simulink model "PLL_fault_no_switching"  (R2022a)
settings: Solver=FixedStepAuto  StartTime=0.0  StopTime=1  FixedStep=Ts  RelTol=1e-3
values from neighbouring files (symbols this model uses):
  C_dc = 2.25    [PLLpara.m]
  Cf1 = 0.01    [PLLpara.m]
  Cf2 = 0.01    [PLLpara.m]
  dt_sag = t_c    [GFMPara.m]    (also in GFMPara_exp.m; PLLpara.m; VFMPara.m; VFMPara_exp.m)
  f_switching = 20e3    (= 20000)    [GFMPara_exp.m]    (also in PLLpara.m = 10000; VFMPara_exp.m)
  Id0 = Id    [PLLpara.m]
  Iq02 = (Ug*cos(asin((Xg*Id+Rg*Iq)/Ug))+Id*Rg-Iq*Xg)*Cf2+Iq    [PLLpara.m]
  ki_pll1 = ki    [PLLpara.m]
  kp_pll1 = kp    [PLLpara.m]
  Lc = 1e-9    (= 1e-09)    [GFMPara.m]    (also in GFMPara_exp.m; PLLpara.m; VFMPara.m; VFMPara_exp.m)
  Lf = 0.0592    [GFMPara.m]    (also in GFMPara_exp.m; PLLpara.m = 0.05; VFMPara.m = 0.05; VFMPara_exp.m = 0.05)
  Lg1 = X1    [PLLpara.m]    (also in VFMPara.m; VFMPara_exp.m)
  Lgg = Xgg    [PLLpara.m]    (also in VFMPara.m; VFMPara_exp.m)
  Rf = 1e-3    (= 0.001)    [PLLpara.m]
  Rg1 = R1    [PLLpara.m]    (also in VFMPara.m; VFMPara_exp.m = 4*R1/5)
  Rgg = Rgg    [PLLpara.m]    (also in VFMPara.m; VFMPara_exp.m)
  Sbase = 1    [GFMPara.m]    (also in GFMPara_exp.m; PLLpara.m; VFMPara.m; VFMPara_exp.m)
  t0 = t_sim_start +t_start    [PLLpara.m]    (also in VFMPara_exp.m)
  t0_sag = t_sim_start +t_start    [GFMPara.m]    (also in GFMPara_exp.m; PLLpara.m = 20; VFMPara.m; VFMPara_exp.m = 20)
  Tc = 1/f_switching    (= 5e-05)    [GFMPara_exp.m]    (also in PLLpara.m = 0.0001; VFMPara_exp.m)
  tc = t_c    [PLLpara.m]    (also in VFMPara_exp.m)
  Ts = 1/Fs    (= 1e-05)    [GFMPara.m]    (also in GFMPara_exp.m = 1e-06; PLLpara.m = 1e-06; VFMPara.m = 5e-06; VFMPara_exp.m = 1e-06)
  v_sag = Ug_fault    [GFMPara.m]    (also in GFMPara_exp.m; PLLpara.m; VFMPara.m; VFMPara_exp.m)
  Vbase = 1    [GFMPara.m]    (also in GFMPara_exp.m; PLLpara.m; VFMPara.m; VFMPara_exp.m)
  Vdc = 2.5    [PLLpara.m]
  w_i_GFL1 = 3000 *2*pi    (= 18849.5559215)    [PLLpara.m]
  w_i_GFL2 = 1100 *2*pi    (= 6911.5038379)    [PLLpara.m]
  w_pll1 = 10 *2*pi    (= 62.8318530718)    [PLLpara.m]
  w_tau1 = 1500 *2*pi    (= 9424.77796077)    [PLLpara.m]
  Wbase = 2*pi*50    (= 314.159265359)    [GFMPara.m]    (also in GFMPara_exp.m; PLLpara.m; VFMPara.m; VFMPara_exp.m)
  Zbase = Vbase/Ibase    (= 1)    [GFMPara.m]    (also in GFMPara_exp.m; PLLpara.m; VFMPara.m; VFMPara_exp.m)
undefined symbols (not defined in the file or in its folder): DiscIntNeverNeededParam, Id, initial, Iq, position, postfault_SEP, w_max, w_min, Ws
libraries: spsVoltageMeasurementLib x52, spsCurrentMeasurementLib x48, spsThreePhaseSeriesRLCBranchLib x13, spsControlledVoltageSourceLib x12, powerlib_extras x12, spsIdealSwitchLib x12, spsSeriesRLCBranchLib x7, spsThreePhaseBreakerLib x4, spsHalfBridgeConverterLib x3, spsDCVoltageSourceLib x2, spsThreePhaseFaultLib x2, cstblocks x1
(part 2 of 4)

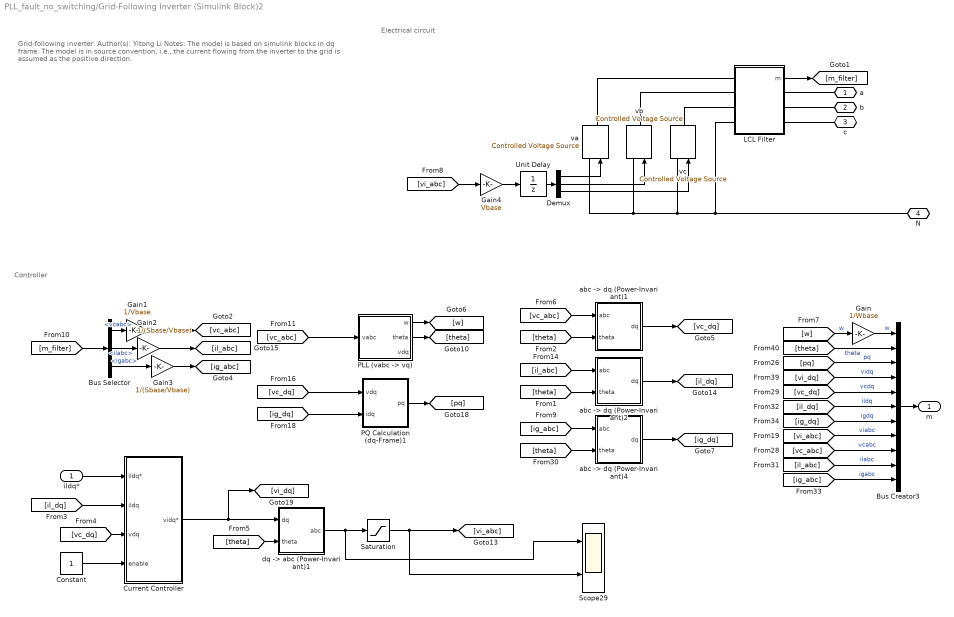
== system PLL_fault_no_switching/Grid-Following Inverter (Simulink Block)2 ==
  note: Grid-following inverter.
      |
      | Author(s): Yitong Li
      |
      | Notes:
      |
      | The model is based on simulink blocks in dq frame.
      |
      | The model is in source convention, i.e., the current flowing from the inverter to the grid is assumed as the positive direction.
  note: Electrical circuit
  note: Controller
  ildq* : Inport
  Bus Creator3 : BusCreator  Inputs=11
  Bus Selector : BusSelector  OutputSignals=vcabc,ilabc,igabc
  Constant : Constant
  Current Controller : Subsystem  mask{Ts=Ts, Wbase=Wbase, Lf=Lf/Wbase, Kg=0, Kp=w_i*Lf/Wbase, Ki=w_i*w_i/4*Lf/Wbase, vdmax=inf, vqmax=inf, Kcd=0}
      mask prompts: Ts "Sampling Time (s)"; Wbase "Base Angular Frequency (rad/s)"; Lf "Inductance"; Kg "Estimator Gain"; Kp "Proportional Gain"; Ki "Integral Gain"; vdmax "Voltage D Limit"; vqmax "Voltage Q Limit"; Kcd "Cross Decoupling Gain"
  Demux : Demux  Outputs=3
  Gain : Gain  Gain=1/Wbase
  Gain1 : Gain  Gain=1/Vbase
  Gain2 : Gain  Gain=1/(Sbase/Vbase)
  Gain3 : Gain  Gain=1/(Sbase/Vbase)
  Gain4 : Gain  Gain=Vbase
  LCL Filter : Subsystem  AncestorBlock=SimplexPS/LCL Filter  mask{Lf=Lf*(Vbase^2/Sbase)/Wbase, Rf=Lf*(Vbase^2/Sbase)/5, Lc=Lc*(Vbase^2/Sbase)/Wbase, Rc=Lc*(Vbase^2/Sbase)/5, Cf=Cf*(Sbase/Vbase^2)/Wbase, Rd=1e-5*(Vbase^2/Sbase)}
      mask prompts: Lf "Lf (H)"; Rf "Rf (Ohm)"; Lc "Lc (H)"; Rc "Rc (Ohm)"; Cf "Cf (F)"; Rd "Rd (Ohm)"
  "PLL (vabc -> vq)" : Subsystem  AncestorBlock=|  mask{Ts=Ts, Vbase=Vbase, Wbase=Wbase, kp=kp_pll1, ki=ki_pll1, w_tau=w_tau1, theta0=0}
      | SimplusGT/PLL
      | (vabc -> vq)
      mask prompts: Ts "Ts (s), sampling period"; Vbase "Vbase (V), base voltage"; Wbase "Wbase (rad/s), base angular frequency"; kp "PLL Proportional Gain"; ki "PLL Integral Gain"; w_tau "w_tau (rad/s), low-pass filter bandwidth"; theta0 "theta0 (rad), initial angle"
  PQ Calculation (dq-Frame)1 : Subsystem  AncestorBlock=|
      | SimplusGT/PQ Calculation
      | (dq-Frame)
  Saturation : Saturate  UpperLimit=2.5/sqrt(3)  LowerLimit=-2.5/sqrt(3)
  Scope29 : Scope  NumInputPorts=2
  Unit Delay : UnitDelay  SampleTime=-1  HasFrameUpgradeWarning=on
  "abc -> dq (Power-Invariant)1" : Subsystem  AncestorBlock=|
      | SimplusGT/abc -> dq
      | (Power-Invariant)
  "abc -> dq (Power-Invariant)2" : Subsystem  AncestorBlock=|
      | SimplusGT/abc -> dq
      | (Power-Invariant)
  "abc -> dq (Power-Invariant)4" : Subsystem  AncestorBlock=|
      | SimplusGT/abc -> dq
      | (Power-Invariant)
  "dq -> abc (Power-Invariant)1" : Subsystem  AncestorBlock=|
      | SimplusGT/dq -> abc
      | (Power-Invariant)
  va : spsControlledVoltageSourceLib/Controlled Voltage Source  Initialize=on  Source_Type=AC  Amplitude=0  Phase=0  Frequency=0  Measurements=None
  vb : spsControlledVoltageSourceLib/Controlled Voltage Source  Initialize=on  Source_Type=AC  Amplitude=0  Phase=0  Frequency=0  Measurements=None
  vc : spsControlledVoltageSourceLib/Controlled Voltage Source  Initialize=on  Source_Type=AC  Amplitude=0  Phase=0  Frequency=0  Measurements=None
  a : PMIOPort  Side=Right
  b : PMIOPort  Port=2  Side=Right
  c : PMIOPort  Port=3  Side=Right
  N : PMIOPort  Port=4  Side=Right
  m : Outport
  wires:
  [vi_abc] -> Gain4/1
  Gain4/1 -> Unit Delay/1
  Gain3/1 -> [ig_abc]
  Gain2/1 -> [il_abc]
  Gain1/1 -> [vc_abc]
  [ig_abc] -> Bus Creator3/11  "igabc"
  [il_abc] -> Bus Creator3/10  "ilabc"
  [vc_abc] -> Bus Creator3/9  "vcabc"
  [vi_abc] -> Bus Creator3/8  "viabc"
  [ig_dq] -> Bus Creator3/7  "igdq"
  [il_dq] -> Bus Creator3/6  "ildq"
  [vc_dq] -> Bus Creator3/5  "vcdq"
  [vi_dq] -> Bus Creator3/4  "vidq"
  [pq] -> Bus Creator3/3  "pq"
  [theta] -> Bus Creator3/2  "theta"
  Gain/1 -> Bus Creator3/1  "w"
  [w] -> Gain/1  "w"
  Bus Selector/1 -> Gain1/1  "<vcabc>"
  Unit Delay/1 -> Demux/1
  [m_filter] -> Bus Selector/1
  "abc -> dq (Power-Invariant)2"/1(dq) -> [il_dq]
  "abc -> dq (Power-Invariant)4"/1(dq) -> [ig_dq]
  "abc -> dq (Power-Invariant)1"/1(dq) -> [vc_dq]
  [vc_abc] -> "PLL (vabc -> vq)"/1(vabc)
  ildq*/1 -> Current Controller/1(iIdq*)
  [ig_dq] -> PQ Calculation (dq-Frame)1/2(idq)
  PQ Calculation (dq-Frame)1/1(pq) -> [pq]
  [vc_dq] -> PQ Calculation (dq-Frame)1/1(vdq)
  [theta] -> "dq -> abc (Power-Invariant)1"/2(theta)
  Current Controller/1(vidq*) -> [vi_dq], "dq -> abc (Power-Invariant)1"/1(dq)
  [vc_dq] -> Current Controller/3(vdq)
  Constant/1 -> Current Controller/4(enable)
  "PLL (vabc -> vq)"/1(w) -> [w]
  "PLL (vabc -> vq)"/2(theta) -> [theta]
  Bus Selector/2 -> Gain2/1  "<ilabc>"
  Bus Selector/3 -> Gain3/1  "<igabc>"
  [theta] -> "abc -> dq (Power-Invariant)4"/2(theta)
  [ig_abc] -> "abc -> dq (Power-Invariant)4"/1(abc)
  [il_abc] -> "abc -> dq (Power-Invariant)2"/1(abc)
  [vc_abc] -> "abc -> dq (Power-Invariant)1"/1(abc)
  [theta] -> "abc -> dq (Power-Invariant)2"/2(theta)
  [theta] -> "abc -> dq (Power-Invariant)1"/2(theta)
  Demux/3 -> vc/1
  Demux/2 -> vb/1
  Demux/1 -> va/1
  LCL Filter/1(m) -> [m_filter]
  Bus Creator3/1 -> m/1
  "dq -> abc (Power-Invariant)1"/1(abc) -> Scope29/1, Saturation/1
  Saturation/1 -> [vi_abc], Scope29/2
  [il_dq] -> Current Controller/2(iIdq)
  connections:
  LCL Filter/LConn3 -- vc/RConn1
  va/LConn1 -- vb/LConn1 -- vc/LConn1 -- LCL Filter/LConn4 -- N/RConn1
  LCL Filter/RConn3 -- c/RConn1
  LCL Filter/RConn2 -- b/RConn1
  LCL Filter/RConn1 -- a/RConn1
  LCL Filter/LConn1 -- va/RConn1
  LCL Filter/LConn2 -- vb/RConn1

== system PLL_fault_no_switching/Voltage Sag1 ==
  note: Pulse generator
      |
      | Author(s): Yitong Li
  Constant : Constant
  Gain : Gain  Gain=1-Am
  Product : Product
  Step : Step  Time=t0  SampleTime=0
  Step1 : Step  Time=t0+dt  Before=1  After=0  SampleTime=0
  Subtract : Sum  Inputs=+-
  Out : Outport
  wires:
  Step1/1 -> Product/2
  Step/1 -> Product/1
  Product/1 -> Gain/1
  Gain/1 -> Subtract/2
  Subtract/1 -> Out/1
  Constant/1 -> Subtract/1

== system PLL_fault_no_switching/Voltage Sag2 ==
  note: Pulse generator
      |
      | Author(s): Yitong Li
  Constant : Constant
  Gain : Gain  Gain=1-Am
  Product : Product
  Step : Step  Time=t0  SampleTime=0
  Step1 : Step  Time=t0+dt  Before=1  After=0  SampleTime=0
  Subtract : Sum  Inputs=+-
  Out : Outport
  wires:
  Step1/1 -> Product/2
  Step/1 -> Product/1
  Product/1 -> Gain/1
  Gain/1 -> Subtract/2
  Subtract/1 -> Out/1
  Constant/1 -> Subtract/1

== system PLL_fault_no_switching/measurement1 ==
  Mux1 : Mux  Inputs=3
  Mux2 : Mux  Inputs=3
  ila : spsCurrentMeasurementLib/Current Measurement  PhasorSimulation=off  OutputType=Complex  PSBequivalent=0
  ilb : spsCurrentMeasurementLib/Current Measurement  PhasorSimulation=off  OutputType=Complex  PSBequivalent=0
  ilc : spsCurrentMeasurementLib/Current Measurement  PhasorSimulation=off  OutputType=Complex  PSBequivalent=0
  vca measure : spsVoltageMeasurementLib/Voltage Measurement  PhasorSimulation=off  OutputType=Complex  PSBequivalent=0
  vcb measure : spsVoltageMeasurementLib/Voltage Measurement  PhasorSimulation=off  OutputType=Complex  PSBequivalent=0
  vcc measure : spsVoltageMeasurementLib/Voltage Measurement  PhasorSimulation=off  OutputType=Complex  PSBequivalent=0
  a : PMIOPort  Side=Left
  b : PMIOPort  Port=2  Side=Left
  c : PMIOPort  Port=3  Side=Left
  n : PMIOPort  Port=4  Side=Left
  A : PMIOPort  Port=5  Side=Right
  B : PMIOPort  Port=6  Side=Right
  C : PMIOPort  Port=7  Side=Right
  N : PMIOPort  Port=8  Side=Right
  Iabc : Outport
  Vabc : Outport  Port=2
  wires:
  ila/1 -> Mux2/1
  ilb/1 -> Mux2/2
  ilc/1 -> Mux2/3
  Mux2/1 -> Iabc/1
  vcb measure/1 -> Mux1/2
  vca measure/1 -> Mux1/1
  vcc measure/1 -> Mux1/3
  Mux1/1 -> Vabc/1
  connections:
  a/RConn1 -- ila/LConn1
  ila/RConn1 -- A/RConn1 -- vca measure/LConn1
  ilb/LConn1 -- b/RConn1
  ilb/RConn1 -- B/RConn1 -- vcb measure/LConn1
  c/RConn1 -- ilc/LConn1
  C/RConn1 -- ilc/RConn1 -- vcc measure/LConn1
  n/RConn1 -- vcc measure/LConn2 -- vcb measure/LConn2 -- vca measure/LConn2 -- N/RConn1

== system PLL_fault_no_switching/measurement10 ==
  Mux1 : Mux  Inputs=3
  Mux2 : Mux  Inputs=3
  ila : spsCurrentMeasurementLib/Current Measurement  PhasorSimulation=off  OutputType=Complex  PSBequivalent=0
  ilb : spsCurrentMeasurementLib/Current Measurement  PhasorSimulation=off  OutputType=Complex  PSBequivalent=0
  ilc : spsCurrentMeasurementLib/Current Measurement  PhasorSimulation=off  OutputType=Complex  PSBequivalent=0
  vca measure : spsVoltageMeasurementLib/Voltage Measurement  PhasorSimulation=off  OutputType=Complex  PSBequivalent=0
  vcb measure : spsVoltageMeasurementLib/Voltage Measurement  PhasorSimulation=off  OutputType=Complex  PSBequivalent=0
  vcc measure : spsVoltageMeasurementLib/Voltage Measurement  PhasorSimulation=off  OutputType=Complex  PSBequivalent=0
  a : PMIOPort  Side=Left
  b : PMIOPort  Port=2  Side=Left
  c : PMIOPort  Port=3  Side=Left
  n : PMIOPort  Port=4  Side=Left
  A : PMIOPort  Port=5  Side=Right
  B : PMIOPort  Port=6  Side=Right
  C : PMIOPort  Port=7  Side=Right
  N : PMIOPort  Port=8  Side=Right
  Iabc : Outport
  Vabc : Outport  Port=2
  wires:
  ila/1 -> Mux2/1
  ilb/1 -> Mux2/2
  ilc/1 -> Mux2/3
  Mux2/1 -> Iabc/1
  vcb measure/1 -> Mux1/2
  vca measure/1 -> Mux1/1
  vcc measure/1 -> Mux1/3
  Mux1/1 -> Vabc/1
  connections:
  a/RConn1 -- ila/LConn1
  ila/RConn1 -- A/RConn1 -- vca measure/LConn1
  ilb/LConn1 -- b/RConn1
  ilb/RConn1 -- B/RConn1 -- vcb measure/LConn1
  c/RConn1 -- ilc/LConn1
  C/RConn1 -- ilc/RConn1 -- vcc measure/LConn1
  n/RConn1 -- vcc measure/LConn2 -- vcb measure/LConn2 -- vca measure/LConn2 -- N/RConn1

== system PLL_fault_no_switching/measurement2 ==
  Mux1 : Mux  Inputs=3
  Mux2 : Mux  Inputs=3
  ila : spsCurrentMeasurementLib/Current Measurement  PhasorSimulation=off  OutputType=Complex  PSBequivalent=0
  ilb : spsCurrentMeasurementLib/Current Measurement  PhasorSimulation=off  OutputType=Complex  PSBequivalent=0
  ilc : spsCurrentMeasurementLib/Current Measurement  PhasorSimulation=off  OutputType=Complex  PSBequivalent=0
  vca measure : spsVoltageMeasurementLib/Voltage Measurement  PhasorSimulation=off  OutputType=Complex  PSBequivalent=0
  vcb measure : spsVoltageMeasurementLib/Voltage Measurement  PhasorSimulation=off  OutputType=Complex  PSBequivalent=0
  vcc measure : spsVoltageMeasurementLib/Voltage Measurement  PhasorSimulation=off  OutputType=Complex  PSBequivalent=0
  a : PMIOPort  Side=Left
  b : PMIOPort  Port=2  Side=Left
  c : PMIOPort  Port=3  Side=Left
  n : PMIOPort  Port=4  Side=Left
  A : PMIOPort  Port=5  Side=Right
  B : PMIOPort  Port=6  Side=Right
  C : PMIOPort  Port=7  Side=Right
  N : PMIOPort  Port=8  Side=Right
  Iabc : Outport
  Vabc : Outport  Port=2
  wires:
  ila/1 -> Mux2/1
  ilb/1 -> Mux2/2
  ilc/1 -> Mux2/3
  Mux2/1 -> Iabc/1
  vcb measure/1 -> Mux1/2
  vca measure/1 -> Mux1/1
  vcc measure/1 -> Mux1/3
  Mux1/1 -> Vabc/1
  connections:
  a/RConn1 -- ila/LConn1
  ila/RConn1 -- A/RConn1 -- vca measure/LConn1
  ilb/LConn1 -- b/RConn1
  ilb/RConn1 -- B/RConn1 -- vcb measure/LConn1
  c/RConn1 -- ilc/LConn1
  C/RConn1 -- ilc/RConn1 -- vcc measure/LConn1
  n/RConn1 -- vcc measure/LConn2 -- vcb measure/LConn2 -- vca measure/LConn2 -- N/RConn1

== system PLL_fault_no_switching/measurement3 ==
  Mux1 : Mux  Inputs=3
  Mux2 : Mux  Inputs=3
  ila : spsCurrentMeasurementLib/Current Measurement  PhasorSimulation=off  OutputType=Complex  PSBequivalent=0
  ilb : spsCurrentMeasurementLib/Current Measurement  PhasorSimulation=off  OutputType=Complex  PSBequivalent=0
  ilc : spsCurrentMeasurementLib/Current Measurement  PhasorSimulation=off  OutputType=Complex  PSBequivalent=0
  vca measure : spsVoltageMeasurementLib/Voltage Measurement  PhasorSimulation=off  OutputType=Complex  PSBequivalent=0
  vcb measure : spsVoltageMeasurementLib/Voltage Measurement  PhasorSimulation=off  OutputType=Complex  PSBequivalent=0
  vcc measure : spsVoltageMeasurementLib/Voltage Measurement  PhasorSimulation=off  OutputType=Complex  PSBequivalent=0
  a : PMIOPort  Side=Left
  b : PMIOPort  Port=2  Side=Left
  c : PMIOPort  Port=3  Side=Left
  n : PMIOPort  Port=4  Side=Left
  A : PMIOPort  Port=5  Side=Right
  B : PMIOPort  Port=6  Side=Right
  C : PMIOPort  Port=7  Side=Right
  N : PMIOPort  Port=8  Side=Right
  Iabc : Outport
  Vabc : Outport  Port=2
  wires:
  ila/1 -> Mux2/1
  ilb/1 -> Mux2/2
  ilc/1 -> Mux2/3
  Mux2/1 -> Iabc/1
  vcb measure/1 -> Mux1/2
  vca measure/1 -> Mux1/1
  vcc measure/1 -> Mux1/3
  Mux1/1 -> Vabc/1
  connections:
  a/RConn1 -- ila/LConn1
  ila/RConn1 -- A/RConn1 -- vca measure/LConn1
  ilb/LConn1 -- b/RConn1
  ilb/RConn1 -- B/RConn1 -- vcb measure/LConn1
  c/RConn1 -- ilc/LConn1
  C/RConn1 -- ilc/RConn1 -- vcc measure/LConn1
  n/RConn1 -- vcc measure/LConn2 -- vcb measure/LConn2 -- vca measure/LConn2 -- N/RConn1

== system PLL_fault_no_switching/measurement4 ==
  Mux1 : Mux  Inputs=3
  Mux2 : Mux  Inputs=3
  ila : spsCurrentMeasurementLib/Current Measurement  PhasorSimulation=off  OutputType=Complex  PSBequivalent=0
  ilb : spsCurrentMeasurementLib/Current Measurement  PhasorSimulation=off  OutputType=Complex  PSBequivalent=0
  ilc : spsCurrentMeasurementLib/Current Measurement  PhasorSimulation=off  OutputType=Complex  PSBequivalent=0
  vca measure : spsVoltageMeasurementLib/Voltage Measurement  PhasorSimulation=off  OutputType=Complex  PSBequivalent=0
  vcb measure : spsVoltageMeasurementLib/Voltage Measurement  PhasorSimulation=off  OutputType=Complex  PSBequivalent=0
  vcc measure : spsVoltageMeasurementLib/Voltage Measurement  PhasorSimulation=off  OutputType=Complex  PSBequivalent=0
  a : PMIOPort  Side=Left
  b : PMIOPort  Port=2  Side=Left
  c : PMIOPort  Port=3  Side=Left
  n : PMIOPort  Port=4  Side=Left
  A : PMIOPort  Port=5  Side=Right
  B : PMIOPort  Port=6  Side=Right
  C : PMIOPort  Port=7  Side=Right
  N : PMIOPort  Port=8  Side=Right
  Iabc : Outport
  Vabc : Outport  Port=2
  wires:
  ila/1 -> Mux2/1
  ilb/1 -> Mux2/2
  ilc/1 -> Mux2/3
  Mux2/1 -> Iabc/1
  vcb measure/1 -> Mux1/2
  vca measure/1 -> Mux1/1
  vcc measure/1 -> Mux1/3
  Mux1/1 -> Vabc/1
  connections:
  a/RConn1 -- ila/LConn1
  ila/RConn1 -- A/RConn1 -- vca measure/LConn1
  ilb/LConn1 -- b/RConn1
  ilb/RConn1 -- B/RConn1 -- vcb measure/LConn1
  c/RConn1 -- ilc/LConn1
  C/RConn1 -- ilc/RConn1 -- vcc measure/LConn1
  n/RConn1 -- vcc measure/LConn2 -- vcb measure/LConn2 -- vca measure/LConn2 -- N/RConn1

== system PLL_fault_no_switching/measurement5 ==
  Mux1 : Mux  Inputs=3
  Mux2 : Mux  Inputs=3
  ila : spsCurrentMeasurementLib/Current Measurement  PhasorSimulation=off  OutputType=Complex  PSBequivalent=0
  ilb : spsCurrentMeasurementLib/Current Measurement  PhasorSimulation=off  OutputType=Complex  PSBequivalent=0
  ilc : spsCurrentMeasurementLib/Current Measurement  PhasorSimulation=off  OutputType=Complex  PSBequivalent=0
  vca measure : spsVoltageMeasurementLib/Voltage Measurement  PhasorSimulation=off  OutputType=Complex  PSBequivalent=0
  vcb measure : spsVoltageMeasurementLib/Voltage Measurement  PhasorSimulation=off  OutputType=Complex  PSBequivalent=0
  vcc measure : spsVoltageMeasurementLib/Voltage Measurement  PhasorSimulation=off  OutputType=Complex  PSBequivalent=0
  a : PMIOPort  Side=Left
  b : PMIOPort  Port=2  Side=Left
  c : PMIOPort  Port=3  Side=Left
  n : PMIOPort  Port=4  Side=Left
  A : PMIOPort  Port=5  Side=Right
  B : PMIOPort  Port=6  Side=Right
  C : PMIOPort  Port=7  Side=Right
  N : PMIOPort  Port=8  Side=Right
  Iabc : Outport
  Vabc : Outport  Port=2
  wires:
  ila/1 -> Mux2/1
  ilb/1 -> Mux2/2
  ilc/1 -> Mux2/3
  Mux2/1 -> Iabc/1
  vcb measure/1 -> Mux1/2
  vca measure/1 -> Mux1/1
  vcc measure/1 -> Mux1/3
  Mux1/1 -> Vabc/1
  connections:
  a/RConn1 -- ila/LConn1
  ila/RConn1 -- A/RConn1 -- vca measure/LConn1
  ilb/LConn1 -- b/RConn1
  ilb/RConn1 -- B/RConn1 -- vcb measure/LConn1
  c/RConn1 -- ilc/LConn1
  C/RConn1 -- ilc/RConn1 -- vcc measure/LConn1
  n/RConn1 -- vcc measure/LConn2 -- vcb measure/LConn2 -- vca measure/LConn2 -- N/RConn1

== system PLL_fault_no_switching/measurement6 ==
  Mux1 : Mux  Inputs=3
  Mux2 : Mux  Inputs=3
  ila : spsCurrentMeasurementLib/Current Measurement  PhasorSimulation=off  OutputType=Complex  PSBequivalent=0
  ilb : spsCurrentMeasurementLib/Current Measurement  PhasorSimulation=off  OutputType=Complex  PSBequivalent=0
  ilc : spsCurrentMeasurementLib/Current Measurement  PhasorSimulation=off  OutputType=Complex  PSBequivalent=0
  vca measure : spsVoltageMeasurementLib/Voltage Measurement  PhasorSimulation=off  OutputType=Complex  PSBequivalent=0
  vcb measure : spsVoltageMeasurementLib/Voltage Measurement  PhasorSimulation=off  OutputType=Complex  PSBequivalent=0
  vcc measure : spsVoltageMeasurementLib/Voltage Measurement  PhasorSimulation=off  OutputType=Complex  PSBequivalent=0
  a : PMIOPort  Side=Left
  b : PMIOPort  Port=2  Side=Left
  c : PMIOPort  Port=3  Side=Left
  n : PMIOPort  Port=4  Side=Left
  A : PMIOPort  Port=5  Side=Right
  B : PMIOPort  Port=6  Side=Right
  C : PMIOPort  Port=7  Side=Right
  N : PMIOPort  Port=8  Side=Right
  Iabc : Outport
  Vabc : Outport  Port=2
  wires:
  ila/1 -> Mux2/1
  ilb/1 -> Mux2/2
  ilc/1 -> Mux2/3
  Mux2/1 -> Iabc/1
  vcb measure/1 -> Mux1/2
  vca measure/1 -> Mux1/1
  vcc measure/1 -> Mux1/3
  Mux1/1 -> Vabc/1
  connections:
  a/RConn1 -- ila/LConn1
  ila/RConn1 -- A/RConn1 -- vca measure/LConn1
  ilb/LConn1 -- b/RConn1
  ilb/RConn1 -- B/RConn1 -- vcb measure/LConn1
  c/RConn1 -- ilc/LConn1
  C/RConn1 -- ilc/RConn1 -- vcc measure/LConn1
  n/RConn1 -- vcc measure/LConn2 -- vcb measure/LConn2 -- vca measure/LConn2 -- N/RConn1

== system PLL_fault_no_switching/measurement7 ==
  Mux1 : Mux  Inputs=3
  Mux2 : Mux  Inputs=3
  ila : spsCurrentMeasurementLib/Current Measurement  PhasorSimulation=off  OutputType=Complex  PSBequivalent=0
  ilb : spsCurrentMeasurementLib/Current Measurement  PhasorSimulation=off  OutputType=Complex  PSBequivalent=0
  ilc : spsCurrentMeasurementLib/Current Measurement  PhasorSimulation=off  OutputType=Complex  PSBequivalent=0
  vca measure : spsVoltageMeasurementLib/Voltage Measurement  PhasorSimulation=off  OutputType=Complex  PSBequivalent=0
  vcb measure : spsVoltageMeasurementLib/Voltage Measurement  PhasorSimulation=off  OutputType=Complex  PSBequivalent=0
  vcc measure : spsVoltageMeasurementLib/Voltage Measurement  PhasorSimulation=off  OutputType=Complex  PSBequivalent=0
  a : PMIOPort  Side=Left
  b : PMIOPort  Port=2  Side=Left
  c : PMIOPort  Port=3  Side=Left
  n : PMIOPort  Port=4  Side=Left
  A : PMIOPort  Port=5  Side=Right
  B : PMIOPort  Port=6  Side=Right
  C : PMIOPort  Port=7  Side=Right
  N : PMIOPort  Port=8  Side=Right
  Iabc : Outport
  Vabc : Outport  Port=2
  wires:
  ila/1 -> Mux2/1
  ilb/1 -> Mux2/2
  ilc/1 -> Mux2/3
  Mux2/1 -> Iabc/1
  vcb measure/1 -> Mux1/2
  vca measure/1 -> Mux1/1
  vcc measure/1 -> Mux1/3
  Mux1/1 -> Vabc/1
  connections:
  a/RConn1 -- ila/LConn1
  ila/RConn1 -- A/RConn1 -- vca measure/LConn1
  ilb/LConn1 -- b/RConn1
  ilb/RConn1 -- B/RConn1 -- vcb measure/LConn1
  c/RConn1 -- ilc/LConn1
  C/RConn1 -- ilc/RConn1 -- vcc measure/LConn1
  n/RConn1 -- vcc measure/LConn2 -- vcb measure/LConn2 -- vca measure/LConn2 -- N/RConn1

== system PLL_fault_no_switching/measurement8 ==
  Mux1 : Mux  Inputs=3
  Mux2 : Mux  Inputs=3
  ila : spsCurrentMeasurementLib/Current Measurement  PhasorSimulation=off  OutputType=Complex  PSBequivalent=0
  ilb : spsCurrentMeasurementLib/Current Measurement  PhasorSimulation=off  OutputType=Complex  PSBequivalent=0
  ilc : spsCurrentMeasurementLib/Current Measurement  PhasorSimulation=off  OutputType=Complex  PSBequivalent=0
  vca measure : spsVoltageMeasurementLib/Voltage Measurement  PhasorSimulation=off  OutputType=Complex  PSBequivalent=0
  vcb measure : spsVoltageMeasurementLib/Voltage Measurement  PhasorSimulation=off  OutputType=Complex  PSBequivalent=0
  vcc measure : spsVoltageMeasurementLib/Voltage Measurement  PhasorSimulation=off  OutputType=Complex  PSBequivalent=0
  a : PMIOPort  Side=Left
  b : PMIOPort  Port=2  Side=Left
  c : PMIOPort  Port=3  Side=Left
  n : PMIOPort  Port=4  Side=Left
  A : PMIOPort  Port=5  Side=Right
  B : PMIOPort  Port=6  Side=Right
  C : PMIOPort  Port=7  Side=Right
  N : PMIOPort  Port=8  Side=Right
  Iabc : Outport
  Vabc : Outport  Port=2
  wires:
  ila/1 -> Mux2/1
  ilb/1 -> Mux2/2
  ilc/1 -> Mux2/3
  Mux2/1 -> Iabc/1
  vcb measure/1 -> Mux1/2
  vca measure/1 -> Mux1/1
  vcc measure/1 -> Mux1/3
  Mux1/1 -> Vabc/1
  connections:
  a/RConn1 -- ila/LConn1
  ila/RConn1 -- A/RConn1 -- vca measure/LConn1
  ilb/LConn1 -- b/RConn1
  ilb/RConn1 -- B/RConn1 -- vcb measure/LConn1
  c/RConn1 -- ilc/LConn1
  C/RConn1 -- ilc/RConn1 -- vcc measure/LConn1
  n/RConn1 -- vcc measure/LConn2 -- vcb measure/LConn2 -- vca measure/LConn2 -- N/RConn1

== system PLL_fault_no_switching/measurement9 ==
  Mux1 : Mux  Inputs=3
  Mux2 : Mux  Inputs=3
  ila : spsCurrentMeasurementLib/Current Measurement  PhasorSimulation=off  OutputType=Complex  PSBequivalent=0
  ilb : spsCurrentMeasurementLib/Current Measurement  PhasorSimulation=off  OutputType=Complex  PSBequivalent=0
  ilc : spsCurrentMeasurementLib/Current Measurement  PhasorSimulation=off  OutputType=Complex  PSBequivalent=0
  vca measure : spsVoltageMeasurementLib/Voltage Measurement  PhasorSimulation=off  OutputType=Complex  PSBequivalent=0
  vcb measure : spsVoltageMeasurementLib/Voltage Measurement  PhasorSimulation=off  OutputType=Complex  PSBequivalent=0
  vcc measure : spsVoltageMeasurementLib/Voltage Measurement  PhasorSimulation=off  OutputType=Complex  PSBequivalent=0
  a : PMIOPort  Side=Left
  b : PMIOPort  Port=2  Side=Left
  c : PMIOPort  Port=3  Side=Left
  n : PMIOPort  Port=4  Side=Left
  A : PMIOPort  Port=5  Side=Right
  B : PMIOPort  Port=6  Side=Right
  C : PMIOPort  Port=7  Side=Right
  N : PMIOPort  Port=8  Side=Right
  Iabc : Outport
  Vabc : Outport  Port=2
  wires:
  ila/1 -> Mux2/1
  ilb/1 -> Mux2/2
  ilc/1 -> Mux2/3
  Mux2/1 -> Iabc/1
  vcb measure/1 -> Mux1/2
  vca measure/1 -> Mux1/1
  vcc measure/1 -> Mux1/3
  Mux1/1 -> Vabc/1
  connections:
  a/RConn1 -- ila/LConn1
  ila/RConn1 -- A/RConn1 -- vca measure/LConn1
  ilb/LConn1 -- b/RConn1
  ilb/RConn1 -- B/RConn1 -- vcb measure/LConn1
  c/RConn1 -- ilc/LConn1
  C/RConn1 -- ilc/RConn1 -- vcc measure/LConn1
  n/RConn1 -- vcc measure/LConn2 -- vcb measure/LConn2 -- vca measure/LConn2 -- N/RConn1

== system PLL_fault_no_switching/AC Infinite Bus (Voltage Type)1/PQ Calculation (dq-Frame)1 ==
  note: Power calculation.
      |
      | Author(s): Yitong Li
      |
      | Notes:
      |
      | The calculation is done in dq frame.
  vdq : Inport
  idq : Inport  Port=2
  Mux : Mux  Inputs=2
  Mux1 : Mux  Inputs=2
  P = vd*id+vq*iq : Fcn  Expr=u[1]*u[3]+u[2]*u[4]
  Q = -vd*iq+vq*id : Fcn  Expr=-u[1]*u[4]+u[2]*u[3]
  pq : Outport
  wires:
  Mux/1 -> pq/1
  P = vd*id+vq*iq/1 -> Mux/1
  vdq/1 -> Mux1/1
  idq/1 -> Mux1/2
  Mux1/1 -> P = vd*id+vq*iq/1, Q = -vd*iq+vq*id/1
  Q = -vd*iq+vq*id/1 -> Mux/2

== system PLL_fault_no_switching/AC Infinite Bus (Voltage Type)1/abc -> dq (Power-Invariant)1 ==
  note: Frame transformation from abc to dq.
      |
      | Author(s): Yitong Li
      |
      | Notes:
      |
      | The transformation is power-invariant.
      |
      | theta is the angle that d axis leads a axis.
      |
      | q axis leads d axis by 90 degrees.
  abc : Inport
  theta : Inport  Port=2
  ->d : Fcn  Expr=cos(u(4))*u(1) + cos(u(4)-2/3*pi)*u(2) + cos(u(4)-4/3*pi)*u(3)
  ->q : Fcn  Expr=-sin(u(4))*u(1) - sin(u(4)-2/3*pi)*u(2) - sin(u(4)-4/3*pi)*u(3)
  Gain : Gain  Gain=sqrt(2/3)
  Mux5 : Mux  Inputs=2
  Mux6 : Mux  Inputs=2
  dq : Outport
  wires:
  abc/1 -> Gain/1
  ->d/1 -> Mux6/1
  Gain/1 -> Mux5/1
  theta/1 -> Mux5/2
  ->q/1 -> Mux6/2
  Mux6/1 -> dq/1
  Mux5/1 -> ->d/1, ->q/1

== system PLL_fault_no_switching/AC Infinite Bus (Voltage Type)1/dq -> abc (Power-Invariant)1 ==
  note: Frame transformation from dq to abc.
      |
      | Author(s): Yitong Li
      |
      | Notes:
      |
      | The transformation is power-invariant.
      |
      | theta is the angle that dq axis leads alpha/beta axis, specifically, d axis leads alpha axis.
  dq : Inport
  theta : Inport  Port=2
  ->a : Fcn  Expr=cos(u(3))*u(1) - sin(u(3))*u(2)
  ->b : Fcn  Expr=cos(u(3)-2/3*pi)*u(1) - sin(u(3)-2/3*pi)*u(2)
  ->c : Fcn  Expr=cos(u(3)-4/3*pi)*u(1) - sin(u(3)-4/3*pi)*u(2)
  Gain : Gain  Gain=sqrt(2/3)
  Mux5 : Mux  Inputs=2
  Mux6 : Mux  Inputs=3
  abc : Outport
  wires:
  ->b/1 -> Mux6/2
  ->a/1 -> Mux6/1
  Gain/1 -> Mux5/1
  dq/1 -> Gain/1
  ->c/1 -> Mux6/3
  Mux6/1 -> abc/1
  Mux5/1 -> ->b/1, ->a/1, ->c/1
  theta/1 -> Mux5/2

== system PLL_fault_no_switching/AC Infinite Bus (Voltage Type)2/PQ Calculation (dq-Frame)1 ==
  note: Power calculation.
      |
      | Author(s): Yitong Li
      |
      | Notes:
      |
      | The calculation is done in dq frame.
  vdq : Inport
  idq : Inport  Port=2
  Mux : Mux  Inputs=2
  Mux1 : Mux  Inputs=2
  P = vd*id+vq*iq : Fcn  Expr=u[1]*u[3]+u[2]*u[4]
  Q = -vd*iq+vq*id : Fcn  Expr=-u[1]*u[4]+u[2]*u[3]
  pq : Outport
  wires:
  Mux/1 -> pq/1
  P = vd*id+vq*iq/1 -> Mux/1
  vdq/1 -> Mux1/1
  idq/1 -> Mux1/2
  Mux1/1 -> P = vd*id+vq*iq/1, Q = -vd*iq+vq*id/1
  Q = -vd*iq+vq*id/1 -> Mux/2

== system PLL_fault_no_switching/AC Infinite Bus (Voltage Type)2/abc -> dq (Power-Invariant)1 ==
  note: Frame transformation from abc to dq.
      |
      | Author(s): Yitong Li
      |
      | Notes:
      |
      | The transformation is power-invariant.
      |
      | theta is the angle that d axis leads a axis.
      |
      | q axis leads d axis by 90 degrees.
  abc : Inport
  theta : Inport  Port=2
  ->d : Fcn  Expr=cos(u(4))*u(1) + cos(u(4)-2/3*pi)*u(2) + cos(u(4)-4/3*pi)*u(3)
  ->q : Fcn  Expr=-sin(u(4))*u(1) - sin(u(4)-2/3*pi)*u(2) - sin(u(4)-4/3*pi)*u(3)
  Gain : Gain  Gain=sqrt(2/3)
  Mux5 : Mux  Inputs=2
  Mux6 : Mux  Inputs=2
  dq : Outport
  wires:
  abc/1 -> Gain/1
  ->d/1 -> Mux6/1
  Gain/1 -> Mux5/1
  theta/1 -> Mux5/2
  ->q/1 -> Mux6/2
  Mux6/1 -> dq/1
  Mux5/1 -> ->d/1, ->q/1

== system PLL_fault_no_switching/AC Infinite Bus (Voltage Type)2/dq -> abc (Power-Invariant)1 ==
  note: Frame transformation from dq to abc.
      |
      | Author(s): Yitong Li
      |
      | Notes:
      |
      | The transformation is power-invariant.
      |
      | theta is the angle that dq axis leads alpha/beta axis, specifically, d axis leads alpha axis.
  dq : Inport
  theta : Inport  Port=2
  ->a : Fcn  Expr=cos(u(3))*u(1) - sin(u(3))*u(2)
  ->b : Fcn  Expr=cos(u(3)-2/3*pi)*u(1) - sin(u(3)-2/3*pi)*u(2)
  ->c : Fcn  Expr=cos(u(3)-4/3*pi)*u(1) - sin(u(3)-4/3*pi)*u(2)
  Gain : Gain  Gain=sqrt(2/3)
  Mux5 : Mux  Inputs=2
  Mux6 : Mux  Inputs=3
  abc : Outport
  wires:
  ->b/1 -> Mux6/2
  ->a/1 -> Mux6/1
  Gain/1 -> Mux5/1
  dq/1 -> Gain/1
  ->c/1 -> Mux6/3
  Mux6/1 -> abc/1
  Mux5/1 -> ->b/1, ->a/1, ->c/1
  theta/1 -> Mux5/2

== system PLL_fault_no_switching/Grid-Following Inverter (Simulink Block)1/Anti-aliasing Filters (7)3 ==
  dq : Inport  PortDimensions=2
  2nd-Order Filter : powerlib_extras/Discrete  Control Blocks/Discrete  2nd-Order Filter  FilterType=Lowpass  Fo=Fc  Zeta=0.707  Ts=Ts  Initialize=off  Vac_Init=[0.8 -25 60]  Vdc_Init=-0.4  PlotResponse=off  param1=[1 2000 0.2]
      settings: SourceProductBaseCode=PS
  2nd-Order Filter1 : powerlib_extras/Discrete  Control Blocks/Discrete  2nd-Order Filter  FilterType=Lowpass  Fo=Fc  Zeta=0.707  Ts=Ts  Initialize=off  Vac_Init=[0.8 -25 60]  Vdc_Init=-0.4  PlotResponse=off  param1=[1 5000 0.1]
      settings: SourceProductBaseCode=PS
  Demux : Demux  Outputs=2
      settings: DisplayOption=none
  Mux : Mux  Inputs=2
  " dq*" : Outport  VectorParamsAs1DForOutWhenUnconnected=off
  wires:
  Demux/2 -> 2nd-Order Filter1/1
  2nd-Order Filter1/1 -> Mux/2
  Mux/1 -> " dq*"/1
  2nd-Order Filter/1 -> Mux/1
  dq/1 -> Demux/1
  Demux/1 -> 2nd-Order Filter/1

== system PLL_fault_no_switching/Grid-Following Inverter (Simulink Block)1/Current Controller ==
  iIdq* : Inport  SampleTime=Tc
  iIdq : Inport  Port=2  SampleTime=Tc
  vdq : Inport  Port=3  SampleTime=Tc
  enable : Inport  Port=4  SampleTime=Tc
  Constant : Constant  Value=Kcd
  Demux1 : Demux  Outputs=2
  Demux2 : Demux  Outputs=2
  Demux3 : Demux  Outputs=2
  Mux : Mux  Inputs=2
  PI-DT-Estimated d : Subsystem  mask{Lf=Lf, Kg=Kg, Kp=Kp, Ki=Ki, xmax=vdmax, xmin=-vdmax, Ts=Ts}
      mask prompts: Lf "Inductance"; Kg "Estimator Gain"; Kp "Proportional Gain"; Ki "Integral Gain"; xmax "Upper Limit"; xmin "Lower Limit"; Ts "Sampling Time"
  PI-DT-Estimated q : Subsystem  mask{Lf=Lf, Kg=Kg, Kp=Kp, Ki=Ki, xmax=vqmax, xmin=-vqmax, Ts=Ts}
      mask prompts: Lf "Inductance"; Kg "Estimator Gain"; Kp "Proportional Gain"; Ki "Integral Gain"; xmax "Upper Limit"; xmin "Lower Limit"; Ts "Sampling Time"
  Product : Product
  Product1 : Product
  sum_d : Sum  Inputs=+-
  sum_q : Sum
  wLd : Gain  Gain=Wbase*Lf
  wLq : Gain  Gain=Wbase*Lf
  vidq* : Outport  SampleTime=Tc
  wires:
  Constant/1 -> Product1/1, Product/2
  Product1/1 -> sum_d/2
  wLq/1 -> Product1/2
  Product/1 -> sum_q/1
  wLd/1 -> Product/1
  enable/1 -> PI-DT-Estimated d/1(enable), PI-DT-Estimated q/4(enable)
  Demux2/2 -> PI-DT-Estimated q/3(reference)
  Demux2/1 -> PI-DT-Estimated d/2(reference)
  iIdq*/1 -> Demux2/1
  Demux3/1 -> PI-DT-Estimated d/3(initial)
  Demux3/2 -> PI-DT-Estimated q/2(initial)
  PI-DT-Estimated q/1(Out) -> sum_q/2
  vdq/1 -> Demux3/1
  PI-DT-Estimated d/1(Out) -> sum_d/1
  Mux/1 -> vidq*/1
  Demux1/2 -> wLq/1, PI-DT-Estimated q/1(actual)
  Demux1/1 -> PI-DT-Estimated d/4(actual), wLd/1
  iIdq/1 -> Demux1/1
  sum_q/1 -> Mux/2
  sum_d/1 -> Mux/1

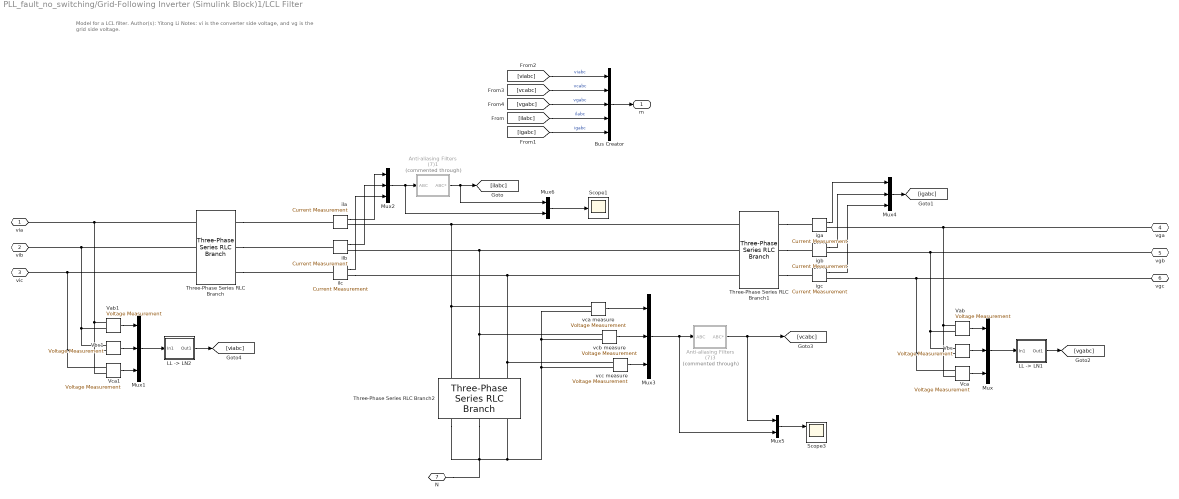
== system PLL_fault_no_switching/Grid-Following Inverter (Simulink Block)1/LCL Filter ==
  note: Model for a LCL filter.
      |
      | Author(s): Yitong Li
      |
      | Notes:
      |
      | vi is the converter side voltage, and vg is the grid side voltage.
  Anti-aliasing Filters (7)1 : Subsystem  Commented=through  mask(Anti-aliasing (2nd order lowpass)){Fc=f_switching, Ts=Ts}
      mask prompts: Fc "Cut-off frequency (Hz):"; Ts "Sample time:"
  Anti-aliasing Filters (7)3 : Subsystem  Commented=through  mask(Anti-aliasing (2nd order lowpass)){Fc=f_switching*2, Ts=Ts}
      mask prompts: Fc "Cut-off frequency (Hz):"; Ts "Sample time:"
  Bus Creator : BusCreator  Inputs=5
  "LL -> LN1" : Subsystem  AncestorBlock=|
      | SimplusGT/Grid-Forming Inverter
      | (Simulink Block)/LCL Filter/LL -> LN1
  "LL -> LN2" : Subsystem  AncestorBlock=|
      | SimplusGT/Grid-Forming Inverter
      | (Simulink Block)/LCL Filter/LL -> LN1
  Mux{,1..4} (5 alike) : Mux  Inputs=3
  Mux5 : Mux  Inputs=2
  Mux6 : Mux  Inputs=2
  Scope1 : Scope
  Scope3 : Scope  NumInputPorts=2
  Three-Phase Series RLC Branch : spsThreePhaseSeriesRLCBranchLib/Three-Phase Series RLC Branch  LConnTagsString=A|B|C  RConnTagsString=A|B|C  BranchType=RL  Resistance=Rf  Inductance=Lf  Capacitance=1e-6  Measurements=None
  Three-Phase Series RLC Branch1 : spsThreePhaseSeriesRLCBranchLib/Three-Phase Series RLC Branch  LConnTagsString=A|B|C  RConnTagsString=A|B|C  BranchType=RL  Resistance=Rc  Inductance=Lc  Capacitance=1e-6  Measurements=None
  Three-Phase Series RLC Branch2 : spsThreePhaseSeriesRLCBranchLib/Three-Phase Series RLC Branch  LConnTagsString=A|B|C  RConnTagsString=A|B|C  BranchType=RC  Resistance=Rd  Inductance=Lc  Capacitance=Cf  Measurements=None
  Vab : spsVoltageMeasurementLib/Voltage Measurement  PhasorSimulation=off  OutputType=Complex  PSBequivalent=0
  Vab1 : spsVoltageMeasurementLib/Voltage Measurement  PhasorSimulation=off  OutputType=Complex  PSBequivalent=0
  Vbc : spsVoltageMeasurementLib/Voltage Measurement  PhasorSimulation=off  OutputType=Complex  PSBequivalent=0
  Vbc1 : spsVoltageMeasurementLib/Voltage Measurement  PhasorSimulation=off  OutputType=Complex  PSBequivalent=0
  Vca : spsVoltageMeasurementLib/Voltage Measurement  PhasorSimulation=off  OutputType=Complex  PSBequivalent=0
  Vca1 : spsVoltageMeasurementLib/Voltage Measurement  PhasorSimulation=off  OutputType=Complex  PSBequivalent=0
  iga : spsCurrentMeasurementLib/Current Measurement  PhasorSimulation=off  OutputType=Complex  PSBequivalent=0
  igb : spsCurrentMeasurementLib/Current Measurement  PhasorSimulation=off  OutputType=Complex  PSBequivalent=0
  igc : spsCurrentMeasurementLib/Current Measurement  PhasorSimulation=off  OutputType=Complex  PSBequivalent=0
  ila : spsCurrentMeasurementLib/Current Measurement  PhasorSimulation=off  OutputType=Complex  PSBequivalent=0
  ilb : spsCurrentMeasurementLib/Current Measurement  PhasorSimulation=off  OutputType=Complex  PSBequivalent=0
  ilc : spsCurrentMeasurementLib/Current Measurement  PhasorSimulation=off  OutputType=Complex  PSBequivalent=0
  vca measure : spsVoltageMeasurementLib/Voltage Measurement  PhasorSimulation=off  OutputType=Complex  PSBequivalent=0
  vcb measure : spsVoltageMeasurementLib/Voltage Measurement  PhasorSimulation=off  OutputType=Complex  PSBequivalent=0
  vcc measure : spsVoltageMeasurementLib/Voltage Measurement  PhasorSimulation=off  OutputType=Complex  PSBequivalent=0
  via : PMIOPort  Side=Left
  vib : PMIOPort  Port=2  Side=Left
  vic : PMIOPort  Port=3  Side=Left
  vga : PMIOPort  Port=4  Side=Right
  vgb : PMIOPort  Port=5  Side=Right
  vgc : PMIOPort  Port=6  Side=Right
  N : PMIOPort  Port=7  Side=Left
  m : Outport
  wires:
  Mux4/1 -> [igabc]
  ilb/1 -> Mux2/2
  ila/1 -> Mux2/1
  igc/1 -> Mux4/3
  vcc measure/1 -> Mux3/3
  Vab/1 -> Mux/1
  Mux/1 -> "LL -> LN1"/1(In1)
  vca measure/1 -> Mux3/1
  vcb measure/1 -> Mux3/2
  igb/1 -> Mux4/2
  iga/1 -> Mux4/1
  Vca/1 -> Mux/3
  ilc/1 -> Mux2/3
  Vbc/1 -> Mux/2
  Bus Creator/1 -> m/1
  "LL -> LN1"/1(Out1) -> [vgabc]
  Vbc1/1 -> Mux1/2
  Vca1/1 -> Mux1/3
  Mux1/1 -> "LL -> LN2"/1(In1)
  Vab1/1 -> Mux1/1
  "LL -> LN2"/1(Out1) -> [viabc]
  [viabc] -> Bus Creator/1  "viabc"
  [vcabc] -> Bus Creator/2  "vcabc"
  [vgabc] -> Bus Creator/3  "vgabc"
  [ilabc] -> Bus Creator/4  "ilabc"
  [igabc] -> Bus Creator/5  "igabc"
  Mux3/1 -> Mux5/2, Anti-aliasing Filters (7)3/1(ABC)
  Anti-aliasing Filters (7)3/1(" ABC*") -> Mux5/1, [vcabc]
  Mux5/1 -> Scope3/1
  Mux6/1 -> Scope1/1
  Anti-aliasing Filters (7)1/1(" ABC*") -> Mux6/1, [ilabc]
  Mux2/1 -> Mux6/2, Anti-aliasing Filters (7)1/1(ABC)
  connections:
  Three-Phase Series RLC Branch2/RConn1 -- Three-Phase Series RLC Branch2/RConn2 -- N/RConn1 -- Three-Phase Series RLC Branch2/RConn3 -- vcc measure/LConn2 -- vca measure/LConn2 -- vcb measure/LConn2
  Vca/LConn1 -- Vbc/LConn2 -- igc/RConn1 -- vgc/RConn1
  Vca1/LConn1 -- Vbc1/LConn2 -- Three-Phase Series RLC Branch/LConn3 -- vic/RConn1
  Vbc1/LConn1 -- Vab1/LConn2 -- vib/RConn1 -- Three-Phase Series RLC Branch/LConn2
  Vab1/LConn1 -- Vca1/LConn2 -- Three-Phase Series RLC Branch/LConn1 -- via/RConn1
  Three-Phase Series RLC Branch1/LConn3 -- ilc/RConn1 -- Three-Phase Series RLC Branch2/LConn3 -- vcc measure/LConn1
  Three-Phase Series RLC Branch1/RConn2 -- igb/LConn1
  Vbc/LConn1 -- Vab/LConn2 -- igb/RConn1 -- vgb/RConn1
  ilb/RConn1 -- Three-Phase Series RLC Branch1/LConn2 -- vcb measure/LConn1 -- Three-Phase Series RLC Branch2/LConn2
  ila/RConn1 -- Three-Phase Series RLC Branch1/LConn1 -- vca measure/LConn1 -- Three-Phase Series RLC Branch2/LConn1
  Vab/LConn1 -- Vca/LConn2 -- iga/RConn1 -- vga/RConn1
  Three-Phase Series RLC Branch1/RConn1 -- iga/LConn1
  Three-Phase Series RLC Branch1/RConn3 -- igc/LConn1
  Three-Phase Series RLC Branch/RConn1 -- ila/LConn1
  Three-Phase Series RLC Branch/RConn2 -- ilb/LConn1
  Three-Phase Series RLC Branch/RConn3 -- ilc/LConn1

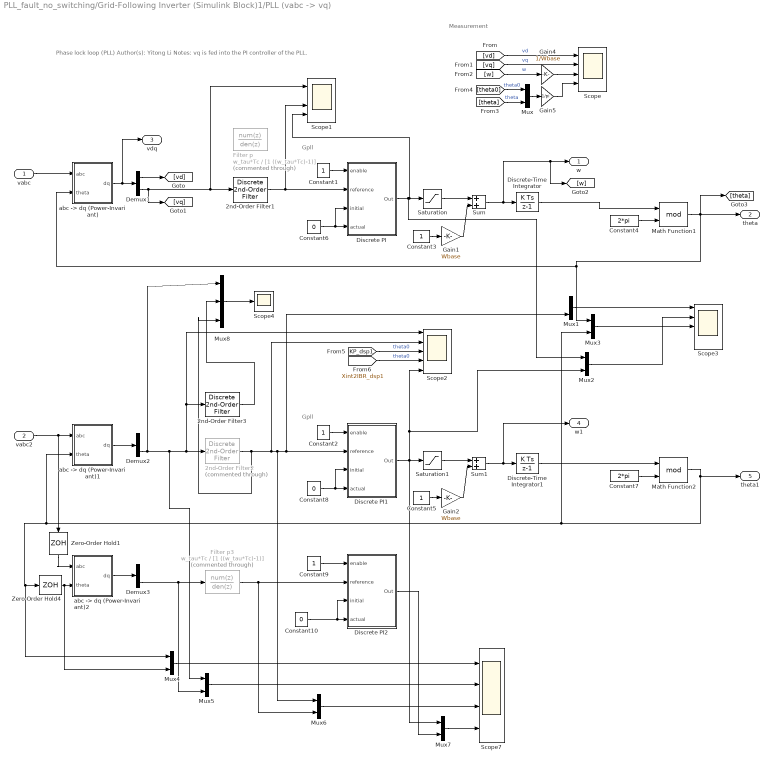
== system PLL_fault_no_switching/Grid-Following Inverter (Simulink Block)1/PLL (vabc -> vq) ==
  note: Measurement
  note: Gpll
  note: Phase lock loop (PLL)
      |
      | Author(s): Yitong Li
      |
      | Notes:
      |
      | vq is fed into the PI controller of the PLL.
  note: Gpll
  vabc : Inport  PortDimensions=3  SampleTime=Tc
  vabc2 : Inport  Port=2  PortDimensions=3  SampleTime=Ts
  2nd-Order Filter1 : powerlib_extras/Discrete  Control Blocks/Discrete  2nd-Order Filter  FilterType=Lowpass  Fo=f_switching/5  Zeta=0.707  Ts=Tc  Initialize=off  Vac_Init=[0.8 -25 60]  Vdc_Init=-0.4  PlotResponse=off  param1=[1 5000 0.1]
      settings: SourceProductBaseCode=PS
  2nd-Order Filter2 : powerlib_extras/Discrete  Control Blocks/Discrete  2nd-Order Filter  Commented=through  FilterType=Lowpass  Fo=f_switching/2  Zeta=0.707  Ts=Ts  Initialize=off  Vac_Init=[0.8 -25 60]  Vdc_Init=-0.4  PlotResponse=off  param1=[1 5000 0.1]
      settings: SourceProductBaseCode=PS
  2nd-Order Filter3 : powerlib_extras/Discrete  Control Blocks/Discrete  2nd-Order Filter  FilterType=Lowpass  Fo=f_switching/2  Zeta=0.707  Ts=Ts  Initialize=off  Vac_Init=[0.8 -25 60]  Vdc_Init=-0.4  PlotResponse=off  param1=[1 5000 0.1]
      settings: SourceProductBaseCode=PS
  Constant{1..3,5,9} (5 alike) : Constant
  Constant10 : Constant  Value=0
  Constant4 : Constant  Value=2*pi
  Constant6 : Constant  Value=0
  Constant7 : Constant  Value=2*pi
  Constant8 : Constant  Value=0
  Demux1 : Demux  Outputs=2
  Demux2 : Demux  Outputs=2
  Demux3 : Demux  Outputs=2
  Discrete PI : Subsystem  AncestorBlock=SimplusGT/Discrete PI  mask{Kp=kp, Ki=ki, xmax=w_max, xmin=w_min, Ts=Tc}
      mask prompts: Kp "Proportional Gain"; Ki "Integral Gain"; xmax "Upper Limit"; xmin "Lower Limit"; Ts "Sampling Time"
  Discrete PI1 : Subsystem  AncestorBlock=SimplusGT/Discrete PI  mask{Kp=kp, Ki=ki, xmax=w_max, xmin=w_min, Ts=Ts}
      mask prompts: Kp "Proportional Gain"; Ki "Integral Gain"; xmax "Upper Limit"; xmin "Lower Limit"; Ts "Sampling Time"
  Discrete PI2 : Subsystem  AncestorBlock=SimplusGT/Discrete PI  mask{Kp=kp, Ki=ki, xmax=w_max, xmin=w_min, Ts=Tc}
      mask prompts: Kp "Proportional Gain"; Ki "Integral Gain"; xmax "Upper Limit"; xmin "Lower Limit"; Ts "Sampling Time"
  Discrete-Time Integrator : DiscreteIntegrator  SampleTime=Tc  ICPrevOutput=DiscIntNeverNeededParam  ICPrevScaledInput=DiscIntNeverNeededParam
  Discrete-Time Integrator1 : DiscreteIntegrator  SampleTime=Ts  ICPrevOutput=DiscIntNeverNeededParam  ICPrevScaledInput=DiscIntNeverNeededParam
  Filter p : DiscreteTransferFcn  Commented=through  Numerator=w_tau*Tc  Denominator=[1 ((w_tau*Tc)-1)]  SampleTime=Tc
  Filter p3 : DiscreteTransferFcn  Commented=through  Numerator=w_tau*Tc  Denominator=[1 ((w_tau*Tc)-1)]  SampleTime=Tc
  Gain1 : Gain  Gain=Wbase
  Gain2 : Gain  Gain=Wbase
  Gain4 : Gain  Gain=1/Wbase
  Gain5 : Gain  Gain=1/pi
  Math Function1 : Math  Operator=mod  SignedPower=on
  Math Function2 : Math  Operator=mod  SignedPower=on
  Mux{,1..7} (8 alike) : Mux  Inputs=2
  Mux8 : Mux  Inputs=3
  Saturation : Saturate  UpperLimit=w_max  LowerLimit=w_min
  Saturation1 : Saturate  UpperLimit=w_max  LowerLimit=w_min
  Scope : Scope  NumInputPorts=4
  Scope1 : Scope  NumInputPorts=4
  Scope2 : Scope  NumInputPorts=5
  Scope3 : Scope  NumInputPorts=5
  Scope4 : Scope
  Scope7 : Scope  NumInputPorts=4
  Sum : Sum
  Sum1 : Sum
  Zero-Order Hold1 : ZeroOrderHold  SampleTime=Tc
  Zero-Order Hold4 : ZeroOrderHold  SampleTime=Tc
  "abc -> dq (Power-Invariant)" : Subsystem  AncestorBlock=|
      | SimplusGT/abc -> dq
      | (Power-Invariant)
  "abc -> dq (Power-Invariant)1" : Subsystem  AncestorBlock=|
      | SimplusGT/abc -> dq
      | (Power-Invariant)
  "abc -> dq (Power-Invariant)2" : Subsystem  AncestorBlock=|
      | SimplusGT/abc -> dq
      | (Power-Invariant)
  w : Outport  SampleTime=Tc
  theta : Outport  Port=2  PortDimensions=1  SampleTime=Tc
  vdq : Outport  Port=3
  w1 : Outport  Port=4  SampleTime=Ts
  theta1 : Outport  Port=5  PortDimensions=1  SampleTime=Ts
  wires:
  vabc/1 -> "abc -> dq (Power-Invariant)"/1(abc)
  "abc -> dq (Power-Invariant)"/1(dq) -> vdq/1, Demux1/1
  Constant4/1 -> Math Function1/2
  Demux1/2 -> Scope1/1, 2nd-Order Filter1/1, [vq]
  Constant6/1 -> Discrete PI/4(actual), Discrete PI/3(initial)
  Constant1/1 -> Discrete PI/1(enable)
  Discrete PI/1(Out) -> Mux2/1, Scope1/4, Saturation/1
  Sum/1 -> [w], w/1, Discrete-Time Integrator/1
  Gain1/1 -> Sum/2
  [vq] -> Scope/2  "vq"
  Mux/1 -> Gain5/1
  Gain4/1 -> Scope/3
  [w] -> Gain4/1  "w"
  [theta0] -> Mux/1  "theta0"
  [vd] -> Scope/1  "vd"
  Gain5/1 -> Scope/4
  [theta] -> Mux/2  "theta"
  Demux1/1 -> [vd]
  Constant3/1 -> Gain1/1
  Math Function1/1 -> "abc -> dq (Power-Invariant)"/2(theta), Mux3/1, [theta], theta/1
  Saturation/1 -> Sum/1
  Math Function2/1 -> theta1/1, Mux3/2, Mux4/1, Zero-Order Hold4/1, "abc -> dq (Power-Invariant)1"/2(theta)
  Saturation1/1 -> Sum1/1
  Constant5/1 -> Gain2/1
  Constant7/1 -> Math Function2/2
  Discrete PI1/1(Out) -> Mux7/1, Mux2/2, Scope2/5, Saturation1/1
  Constant8/1 -> Discrete PI1/4(actual), Discrete PI1/3(initial)
  Demux2/2 -> Mux8/1, Mux5/1, 2nd-Order Filter2/1, 2nd-Order Filter3/1, Scope2/1
  Gain2/1 -> Sum1/2
  Constant2/1 -> Discrete PI1/1(enable)
  vabc2/1 -> Zero-Order Hold1/1, "abc -> dq (Power-Invariant)1"/1(abc)
  Sum1/1 -> w1/1, Discrete-Time Integrator1/1
  2nd-Order Filter2/1 -> Mux8/3, Scope2/2, Mux6/1, Mux1/2, Discrete PI1/2(reference)
  Discrete-Time Integrator1/1 -> Math Function2/1
  "abc -> dq (Power-Invariant)1"/1(dq) -> Demux2/1
  [KP_dsp1] -> Scope2/3  "theta0"
  [Xint2IBR_dsp1] -> Scope2/4  "theta0"
  Mux1/1 -> Scope3/1
  Mux2/1 -> Scope3/2
  Mux3/1 -> Scope3/3
  Zero-Order Hold4/1 -> Mux4/2, "abc -> dq (Power-Invariant)2"/2(theta)
  "abc -> dq (Power-Invariant)2"/1(dq) -> Demux3/1
  Demux3/2 -> Mux5/2, Filter p3/1
  Mux4/1 -> Scope7/1
  Mux5/1 -> Scope7/2
  Mux6/1 -> Scope7/3
  Filter p3/1 -> Discrete PI2/2(reference), Mux6/2
  Zero-Order Hold1/1 -> "abc -> dq (Power-Invariant)2"/1(abc)
  Constant9/1 -> Discrete PI2/1(enable)
  Constant10/1 -> Discrete PI2/4(actual), Discrete PI2/3(initial)
  Mux7/1 -> Scope7/4
  Discrete PI2/1(Out) -> Mux7/2
  2nd-Order Filter3/1 -> Mux8/2
  Mux8/1 -> Scope4/1
  2nd-Order Filter1/1 -> Scope1/3, Discrete PI/2(reference)
  Discrete-Time Integrator/1 -> Math Function1/1

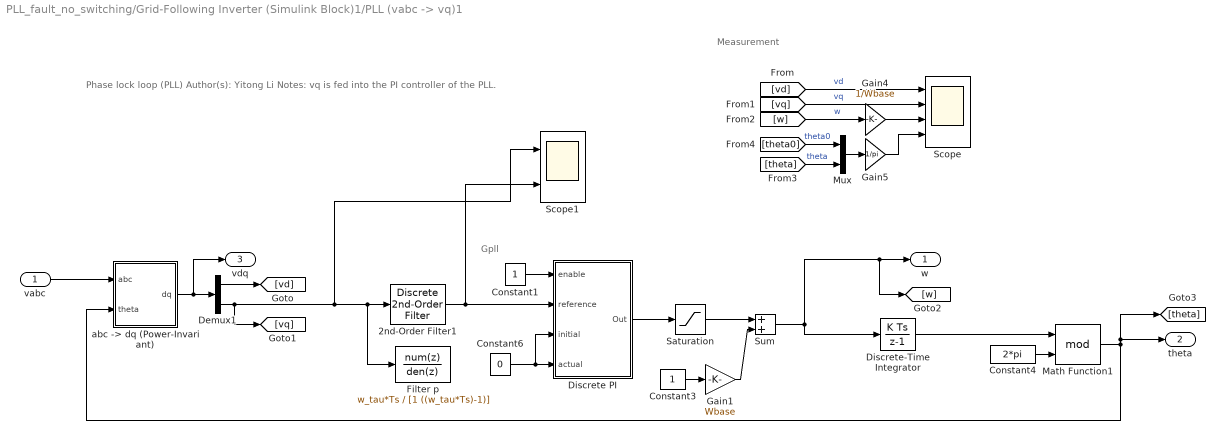
== system PLL_fault_no_switching/Grid-Following Inverter (Simulink Block)1/PLL (vabc -> vq)1 ==
  note: Measurement
  note: Gpll
  note: Phase lock loop (PLL)
      |
      | Author(s): Yitong Li
      |
      | Notes:
      |
      | vq is fed into the PI controller of the PLL.
  vabc : Inport
  2nd-Order Filter1 : powerlib_extras/Discrete  Control Blocks/Discrete  2nd-Order Filter  FilterType=Lowpass  Fo=f_switching/5  Zeta=0.707  Ts=Ts  Initialize=off  Vac_Init=[0.8 -25 60]  Vdc_Init=-0.4  PlotResponse=off  param1=[1 5000 0.1]
      settings: SourceProductBaseCode=PS
  Constant1 : Constant
  Constant3 : Constant
  Constant4 : Constant  Value=2*pi
  Constant6 : Constant  Value=0
  Demux1 : Demux  Outputs=2
  Discrete PI : Subsystem  AncestorBlock=SimplusGT/Discrete PI  mask{Kp=kp, Ki=ki, xmax=w_max, xmin=w_min, Ts=Ts}
      mask prompts: Kp "Proportional Gain"; Ki "Integral Gain"; xmax "Upper Limit"; xmin "Lower Limit"; Ts "Sampling Time"
  Discrete-Time Integrator : DiscreteIntegrator  SampleTime=Ts  ICPrevOutput=DiscIntNeverNeededParam  ICPrevScaledInput=DiscIntNeverNeededParam
  Filter p : DiscreteTransferFcn  Numerator=w_tau*Ts  Denominator=[1 ((w_tau*Ts)-1)]  SampleTime=Ts
  Gain1 : Gain  Gain=Wbase
  Gain4 : Gain  Gain=1/Wbase
  Gain5 : Gain  Gain=1/pi
  Math Function1 : Math  Operator=mod  SignedPower=on
  Mux : Mux  Inputs=2
  Saturation : Saturate  UpperLimit=w_max  LowerLimit=w_min
  Scope : Scope  NumInputPorts=4
  Scope1 : Scope  NumInputPorts=2
  Sum : Sum
  "abc -> dq (Power-Invariant)" : Subsystem  AncestorBlock=|
      | SimplusGT/abc -> dq
      | (Power-Invariant)
  w : Outport
  theta : Outport  Port=2
  vdq : Outport  Port=3
  wires:
  vabc/1 -> "abc -> dq (Power-Invariant)"/1(abc)
  "abc -> dq (Power-Invariant)"/1(dq) -> vdq/1, Demux1/1
  Constant4/1 -> Math Function1/2
  Demux1/2 -> [vq], Scope1/1, 2nd-Order Filter1/1, Filter p/1
  Constant6/1 -> Discrete PI/4(actual), Discrete PI/3(initial)
  Constant1/1 -> Discrete PI/1(enable)
  Discrete PI/1(Out) -> Saturation/1
  Sum/1 -> [w], w/1, Discrete-Time Integrator/1
  Gain1/1 -> Sum/2
  [vq] -> Scope/2  "vq"
  Mux/1 -> Gain5/1
  Gain4/1 -> Scope/3
  [w] -> Gain4/1  "w"
  [theta0] -> Mux/1  "theta0"
  [vd] -> Scope/1  "vd"
  Gain5/1 -> Scope/4
  [theta] -> Mux/2  "theta"
  Demux1/1 -> [vd]
  Constant3/1 -> Gain1/1
  Math Function1/1 -> [theta], theta/1, "abc -> dq (Power-Invariant)"/2(theta)
  Saturation/1 -> Sum/1
  Discrete-Time Integrator/1 -> Math Function1/1
  2nd-Order Filter1/1 -> Scope1/2, Discrete PI/2(reference)

== system PLL_fault_no_switching/Grid-Following Inverter (Simulink Block)1/PQ Calculation (dq-Frame)1 ==
  note: Power calculation.
      |
      | Author(s): Yitong Li
      |
      | Notes:
      |
      | The calculation is done in dq frame.
  vdq : Inport
  idq : Inport  Port=2
  Mux : Mux  Inputs=2
  Mux1 : Mux  Inputs=2
  P = vd*id+vq*iq : Fcn  Expr=u[1]*u[3]+u[2]*u[4]
  Q = -vd*iq+vq*id : Fcn  Expr=-u[1]*u[4]+u[2]*u[3]
  pq : Outport
  wires:
  Mux/1 -> pq/1
  P = vd*id+vq*iq/1 -> Mux/1
  vdq/1 -> Mux1/1
  idq/1 -> Mux1/2
  Mux1/1 -> P = vd*id+vq*iq/1, Q = -vd*iq+vq*id/1
  Q = -vd*iq+vq*id/1 -> Mux/2

== system PLL_fault_no_switching/Grid-Following Inverter (Simulink Block)1/abc -> dq (Power-Invariant)1 ==
  note: Frame transformation from abc to dq.
      |
      | Author(s): Yitong Li
      |
      | Notes:
      |
      | The transformation is power-invariant.
      |
      | theta is the angle that d axis leads a axis.
      |
      | q axis leads d axis by 90 degrees.
  abc : Inport  SampleTime=Tc
  theta : Inport  Port=2  SampleTime=Tc
  ->d : Fcn  Expr=cos(u(4))*u(1) + cos(u(4)-2/3*pi)*u(2) + cos(u(4)-4/3*pi)*u(3)
  ->q : Fcn  Expr=-sin(u(4))*u(1) - sin(u(4)-2/3*pi)*u(2) - sin(u(4)-4/3*pi)*u(3)
  Gain : Gain  Gain=sqrt(2/3)
  Mux5 : Mux  Inputs=2
  Mux6 : Mux  Inputs=2
  dq : Outport  SampleTime=Tc
  wires:
  abc/1 -> Gain/1
  ->d/1 -> Mux6/1
  Gain/1 -> Mux5/1
  theta/1 -> Mux5/2
  ->q/1 -> Mux6/2
  Mux6/1 -> dq/1
  Mux5/1 -> ->d/1, ->q/1

== system PLL_fault_no_switching/Grid-Following Inverter (Simulink Block)1/abc -> dq (Power-Invariant)2 ==
  note: Frame transformation from abc to dq.
      |
      | Author(s): Yitong Li
      |
      | Notes:
      |
      | The transformation is power-invariant.
      |
      | theta is the angle that d axis leads a axis.
      |
      | q axis leads d axis by 90 degrees.
  abc : Inport  SampleTime=Tc
  theta : Inport  Port=2  SampleTime=Tc
  ->d : Fcn  Expr=cos(u(4))*u(1) + cos(u(4)-2/3*pi)*u(2) + cos(u(4)-4/3*pi)*u(3)
  ->q : Fcn  Expr=-sin(u(4))*u(1) - sin(u(4)-2/3*pi)*u(2) - sin(u(4)-4/3*pi)*u(3)
  Gain : Gain  Gain=sqrt(2/3)
  Mux5 : Mux  Inputs=2
  Mux6 : Mux  Inputs=2
  dq : Outport  SampleTime=Tc
  wires:
  abc/1 -> Gain/1
  ->d/1 -> Mux6/1
  Gain/1 -> Mux5/1
  theta/1 -> Mux5/2
  ->q/1 -> Mux6/2
  Mux6/1 -> dq/1
  Mux5/1 -> ->d/1, ->q/1

== system PLL_fault_no_switching/Grid-Following Inverter (Simulink Block)1/abc -> dq (Power-Invariant)3 ==
  note: Frame transformation from abc to dq.
      |
      | Author(s): Yitong Li
      |
      | Notes:
      |
      | The transformation is power-invariant.
      |
      | theta is the angle that d axis leads a axis.
      |
      | q axis leads d axis by 90 degrees.
  abc : Inport  SampleTime=Tc
  theta : Inport  Port=2  SampleTime=Tc
  ->d : Fcn  Expr=cos(u(4))*u(1) + cos(u(4)-2/3*pi)*u(2) + cos(u(4)-4/3*pi)*u(3)
  ->q : Fcn  Expr=-sin(u(4))*u(1) - sin(u(4)-2/3*pi)*u(2) - sin(u(4)-4/3*pi)*u(3)
  Gain : Gain  Gain=sqrt(2/3)
  Mux5 : Mux  Inputs=2
  Mux6 : Mux  Inputs=2
  dq : Outport  SampleTime=Tc
  wires:
  abc/1 -> Gain/1
  ->d/1 -> Mux6/1
  Gain/1 -> Mux5/1
  theta/1 -> Mux5/2
  ->q/1 -> Mux6/2
  Mux6/1 -> dq/1
  Mux5/1 -> ->d/1, ->q/1
